simulink model "H9_Heric_2__new_series_switching_upcoming_conference"  (R2018a)
settings: Solver=ode45  StartTime=0.0  StopTime=.04  RelTol=1e-3  EnableMultiTasking=on
libraries: powerlib x53, powerlib_extras x6, powerlib_meascontrol x5, pePowerMeasurement x1, simulink x1
settings Model: Creator=Personal  LastModifiedBy=HP
settings DataIOCC: LimitDataPoints=on  SaveFormat=Array
settings OptimizationCC: LifeSpan=inf
settings DebuggingCC: SolverPrmCheckMsg=warning  SFUnexpectedBacktrackingDiag=warning  SFNoUnconditionalDefaultTransitionDiag=warning  SFExecutionAtInitializationDiag=none
settings HardwareCC: ProdBitPerPointer=32  ProdBitPerSizeT=32  ProdBitPerPtrDiffT=32  ProdLargestAtomicFloat=None  ProdIntDivRoundTo=Undefined  ProdEndianess=Unspecified  ProdWordSize=32  ProdHWDeviceType=32-bit Generic
settings ModelReferenceCC: PropagateSignalLabelsOutOfModel=off
settings CodeAppCC: StateflowObjectComments=on
settings GRTTargetCC: TargetLangStandard=C89/C90 (ANSI)  GeneratePreprocessorConditionals=Disable all
settings ConfigComp: CovMetricSettings=dw  CovHtmlReporting=on  CovSaveCumulativeToWorkspaceVar=on  CovSaveSingleToWorkspaceVar=on  CovExternalEMLEnable=off  CovSFcnEnable=off
settings SimscapeCC: SimscapeNormalizeSystem=off

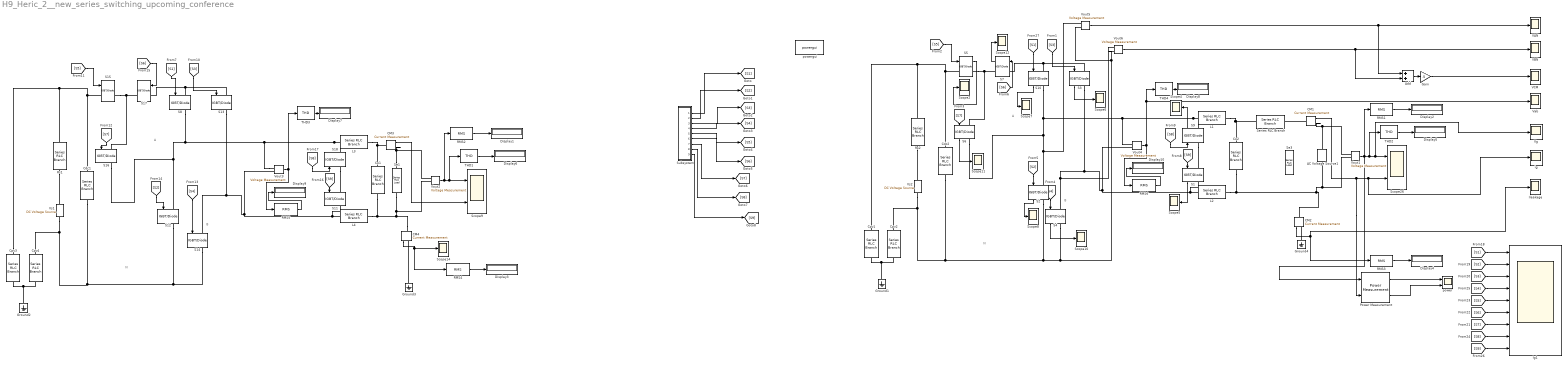
== system H9_Heric_2__new_series_switching_upcoming_conference ==
  note: B
  note: A
  note: N
  note: A
  note: N
  note: B
  AC Voltage Source1 : powerlib/Electrical Sources/AC Voltage Source  Amplitude=220  Phase=0  Frequency=50  SampleTime=0  Measurements=None  BusType=swing  Pref=10e3  Qref=0  Qmin=-inf  Qmax=+inf
  Add : Sum
  CM{1..4} (4 alike) : powerlib/Measurements/Current Measurement  PhasorSimulation=off  OutputType=Complex  PSBequivalent=0
  Cdc1 : powerlib/Elements/Series RLC Branch  LConnTagsString=__new0  RConnTagsString=__new0  BranchType=C  Resistance=1  Inductance=3e-3  SetiL0=off  InitialCurrent=0  Capacitance=940e-6  Setx0=off  InitialVoltage=0  Measurements=None
  Cdc2 : powerlib/Elements/Series RLC Branch  LConnTagsString=__new0  RConnTagsString=__new0  BranchType=C  Resistance=1  Inductance=3e-3  SetiL0=off  InitialCurrent=0  Capacitance=940e-6  Setx0=off  InitialVoltage=0  Measurements=None
  Co1 : powerlib/Elements/Series RLC Branch  LConnTagsString=__new0  RConnTagsString=__new0  BranchType=C  Resistance=1  Inductance=3e-3  SetiL0=off  InitialCurrent=0  Capacitance=2.2e-6  Setx0=off  InitialVoltage=0  Measurements=None
  Co2 : powerlib/Elements/Series RLC Branch  LConnTagsString=__new0  RConnTagsString=__new0  BranchType=C  Resistance=1  Inductance=3e-3  SetiL0=off  InitialCurrent=0  Capacitance=2.2e-6  Setx0=off  InitialVoltage=0  Measurements=None
  Cpv{1..4} (4 alike) : powerlib/Elements/Series RLC Branch  LConnTagsString=__new0  RConnTagsString=__new0  BranchType=C  Resistance=1  Inductance=3e-3  SetiL0=off  InitialCurrent=0  Capacitance=75e-9  Setx0=off  InitialVoltage=0  Measurements=None
  Display{1..10} (10 alike) : Display
  Gain : Gain  Gain=.5
  Ground{1..4} (4 alike) : powerlib/Elements/Ground  LConnTagsString=a
  Ig1 : Scope  NumInputPorts=9
  Ileakage : Scope
  L{1..4} (4 alike) : powerlib/Elements/Series RLC Branch  LConnTagsString=__new0  RConnTagsString=__new0  BranchType=L  Resistance=1  Inductance=3e-3  SetiL0=off  InitialCurrent=0  Capacitance=1e-6  Setx0=off  InitialVoltage=0  Measurements=None
  Power Measurement : pePowerMeasurement/Power Measurement  OverrideUsingVariant=Continuous  F=60  K=[0 1 2 3]  Ts=0
  RMS{1..6} (6 alike) : powerlib_extras/Measurements/RMS  f1=50
  Rs1 : powerlib/Elements/Series RLC Branch  LConnTagsString=__new0  RConnTagsString=__new0  BranchType=R  Resistance=1  Inductance=3e-3  SetiL0=off  InitialCurrent=0  Capacitance=1e-6  Setx0=off  InitialVoltage=0  Measurements=None
  Rs2 : powerlib/Elements/Series RLC Branch  LConnTagsString=__new0  RConnTagsString=__new0  BranchType=R  Resistance=1  Inductance=3e-3  SetiL0=off  InitialCurrent=0  Capacitance=1e-6  Setx0=off  InitialVoltage=0  Measurements=None
  S{1..18} (18 alike) : powerlib/Power Electronics/IGBT//Diode  Ron=1e-3  Rs=1e5  Cs=inf  Measurements=on
  Scope{2,4..8,10..12,14} (10 alike) : Scope
  Scope26 : Scope  NumInputPorts=2
  Scope9 : Scope  NumInputPorts=2
  Se1 : powerlib/Elements/Series RLC Load  LConnTagsString=a  RConnTagsString=__new0  NominalVoltage=230  NominalFrequency=50  ActivePower=1000  InductivePower=0  CapacitivePower=0  Setx0=off  InitialVoltage=0  SetiL0=off  InitialCurrent=0  Measurements=None  LoadType=constant Z
  Se3 : powerlib/Elements/Series RLC Load  LConnTagsString=a  RConnTagsString=__new0  NominalVoltage=230  NominalFrequency=50  ActivePower=1000  InductivePower=0  CapacitivePower=0  Setx0=off  InitialVoltage=0  SetiL0=off  InitialCurrent=0  Measurements=None  LoadType=constant Z
  Series RLC Branch : powerlib/Elements/Series RLC Branch  LConnTagsString=__new0  RConnTagsString=__new0  BranchType=R  Resistance=10  Inductance=1e-3  SetiL0=off  InitialCurrent=0  Capacitance=0  Setx0=off  InitialVoltage=0  Measurements=None
  Subsystem : Subsystem
  THD1 : powerlib_meascontrol/Measurements/THD  Freq=50  Ts=0
  THD2 : powerlib_meascontrol/Measurements/THD  Freq=50  Ts=0
  THD3 : powerlib_meascontrol/Measurements/THD  Freq=60  Ts=0
  THD4 : powerlib_meascontrol/Measurements/THD  Freq=60  Ts=0
  VAN : Scope
  VBN : Scope
  VCM : Scope
  Vab : Scope
  Vg : Scope
  Vout{1..6} (6 alike) : powerlib/Measurements/Voltage Measurement  PhasorSimulation=off  OutputType=Complex  PSBequivalent=0
  Vs1 : powerlib/Electrical Sources/DC Voltage Source  Amplitude=330  Measurements=None
  Vs2 : powerlib/Electrical Sources/DC Voltage Source  Amplitude=330  Measurements=None
  ig : Scope
  power : Scope  NumInputPorts=2
  powergui : powerlib/powergui  Priority=1  SimulationMode=Continuous  SampleTime=50e-6  frequency=60  Iterations=50  frequencyindice=0  Pbase=100e6  ErrMax=1e-4  UnitsV=kV  UnitsW=MW  buscounter=0  FunctionMessages=off  echomessages=off  EnableUseOfTLC=off  CurrentSourceSwitches=off  DisableSnubberDevices=off  DisableRonSwitches=off  DisableVfSwitches=off  DisplayEquations=off  SolverType=Tustin/Backward Euler (TBE)  Interpol=off  ExternalGateDelay=off  methode=off  Ts=100  x0status=blocks  SPID=on  SwTol=0  HookPort=off  RestoreLinks=warning  ResistiveCurrentMeasurement=off  Frange=[0:2:500]  Ylog=off  Xlog=on  ShowGrid=off  save=off  variable=ZData  structure=ig  ZoomFFT=off  StartTime=0.02  cycles=1  DisplayStyle=1  fundamental=50  FreqAxis=off  MaxFrequency=10000  frequencyindicesteady=1  RmsSteady=1  display=off
  wires:
  Subsystem/1(Out1) -> [S1]
  Subsystem/2(Out2) -> [S2]
  Subsystem/3(Out3) -> [S3]
  Subsystem/4(Out4) -> [S4]
  Subsystem/5(Out5) -> [S5]
  Subsystem/6(Out6) -> [S6]
  Subsystem/7(Out7) -> [S7]
  Subsystem/8(Out8) -> [S8]
  Subsystem/9(Out9) -> [S9]
  ? -> ?
  [S5] -> S15/1
  [S8] -> S18/1
  [S6] -> S17/1
  [S9] -> S11/1
  CM3/1 -> Scope9/2
  CM4/1 -> Scope14/1, RMS4/1
  [S7] -> S16/1
  RMS4/1 -> Display3/1
  [S1] -> S8/1
  THD3/1 -> Display7/1
  [S2] -> S12/1
  Vout2/1 -> RMS2/1, THD1/1, Scope9/1
  THD1/1 -> Display6/1
  [S4] -> S14/1
  RMS5/1 -> Display9/1
  RMS2/1 -> Display1/1
  [S3] -> S13/1
  Vout3/1 -> THD3/1, RMS5/1
  [S4] -> Ig1/4
  [S6] -> Ig1/6
  [S5] -> Ig1/5
  [S7] -> Ig1/7
  [S1] -> Ig1/1
  [S3] -> Ig1/3
  [S2] -> Ig1/2
  [S8] -> Ig1/8
  [S9] -> Ig1/9
  RMS6/1 -> Display10/1
  RMS1/1 -> Display2/1
  [S4] -> S4/1
  [S7] -> S6/1
  [S1] -> S10/1
  S3/1 -> Scope6/1
  [S2] -> S2/1
  THD2/1 -> Display5/1
  S2/1 -> Scope8/1
  S9/1 -> Scope4/1
  RMS3/1 -> Display4/1
  Vout4/1 -> THD4/1, Vab/1, RMS6/1
  S6/1 -> Scope11/1
  [S3] -> S3/1
  S10/1 -> Scope7/1
  [S8] -> S9/1
  [S5] -> S5/1
  [S6] -> S7/1
  [S9] -> S1/1
  THD4/1 -> Display8/1
  S7/1 -> Scope12/1
  CM2/1 -> Ileakage/1, RMS3/1
  S4/1 -> Scope10/1
  S5/1 -> Scope2/1
  S1/1 -> Scope5/1
  Vout6/1 -> Add/2, VBN/1
  Vout5/1 -> Add/1, VAN/1
  Add/1 -> Gain/1
  Gain/1 -> VCM/1
  Power Measurement/1 -> power/1
  Vout1/1 -> Scope26/1, Vg/1, THD2/1, RMS1/1, Power Measurement/1
  Power Measurement/2 -> power/2
  CM1/1 -> Power Measurement/2, ig/1, Scope26/2
  connections:
  S12/RConn1 -- S14/RConn1 -- Vs1/LConn1 -- Cpv4/LConn1 -- Cdc1/RConn1
  S17/LConn1 -- S13/LConn1 -- S8/LConn1
  S13/RConn1 -- Vout3/LConn2 -- L4/LConn1 -- S11/RConn1 -- S14/LConn1
  CM4/LConn1 -- Vout2/LConn2 -- Se1/RConn1 -- L4/RConn1 -- Co1/RConn1
  Cpv3/LConn1 -- Cdc1/LConn1 -- S15/LConn1 -- Rs1/RConn1
  Vout3/LConn1 -- S16/RConn1 -- S12/LConn1 -- S8/RConn1 -- L3/LConn1 -- S18/RConn1
  Co1/LConn1 -- L3/RConn1 -- CM3/LConn1
  S16/LConn1 -- S15/RConn1 -- S17/RConn1
  Cpv3/RConn1 -- Ground2/LConn1 -- Cpv4/RConn1
  Se1/LConn1 -- CM3/RConn1 -- Vout2/LConn1
  Ground3/LConn1 -- CM4/RConn1
  Rs1/LConn1 -- Vs1/RConn1
  S18/LConn1 -- S11/LConn1
  S9/RConn1 -- Vout4/LConn1 -- S6/RConn1 -- S2/LConn1 -- Vout5/LConn1 -- S10/RConn1 -- L1/LConn1
  Cpv2/RConn1 -- Cpv1/RConn1 -- Ground1/LConn1
  Vout1/LConn2 -- CM2/LConn1 -- L2/RConn1 -- Co2/RConn1 -- AC Voltage Source1/LConn1
  S5/LConn1 -- Cpv1/LConn1 -- Rs2/RConn1 -- Cdc2/LConn1
  S10/LConn1 -- S7/LConn1 -- S3/LConn1
  S4/RConn1 -- Vout6/LConn2 -- Vout5/LConn2 -- Vs2/LConn1 -- Cpv2/LConn1 -- Cdc2/RConn1 -- S2/RConn1
  S1/RConn1 -- S4/LConn1 -- Vout6/LConn1 -- S3/RConn1 -- Vout4/LConn2 -- L2/LConn1
  CM1/LConn1 -- Series RLC Branch/RConn1
  Vout1/LConn1 -- CM1/RConn1 -- AC Voltage Source1/RConn1
  S7/RConn1 -- S6/LConn1 -- S5/RConn1
  Ground4/LConn1 -- CM2/RConn1
  Rs2/LConn1 -- Vs2/RConn1
  S9/LConn1 -- S1/LConn1
  Series RLC Branch/LConn1 -- Co2/LConn1 -- L1/RConn1

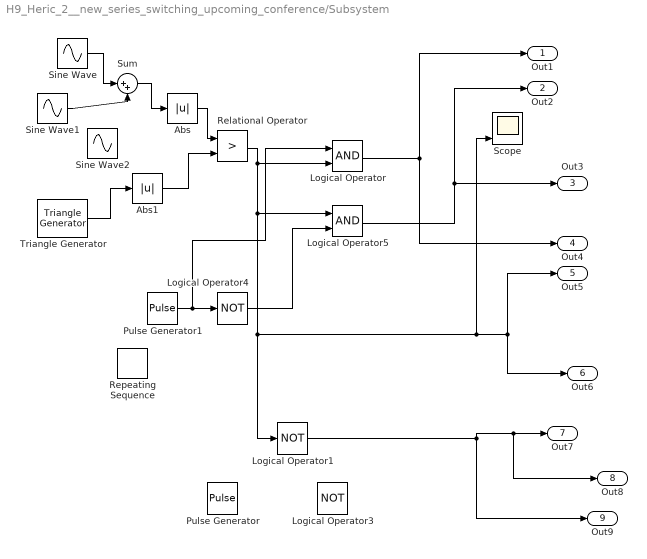
== system H9_Heric_2__new_series_switching_upcoming_conference/Subsystem ==
  Abs : Abs
  Abs1 : Abs
  Logical Operator : Logic  AllPortsSameDT=off  OutDataTypeStr=boolean
  Logical Operator1 : Logic  Operator=NOT  AllPortsSameDT=off  OutDataTypeStr=boolean
  Logical Operator3 : Logic  Operator=NOT  AllPortsSameDT=off  OutDataTypeStr=boolean
  Logical Operator4 : Logic  Operator=NOT  AllPortsSameDT=off  OutDataTypeStr=boolean
  Logical Operator5 : Logic  AllPortsSameDT=off  OutDataTypeStr=boolean
  Pulse Generator : DiscretePulseGenerator  PulseType=Time based  Period=.02  PulseWidth=50
  Pulse Generator1 : DiscretePulseGenerator  PulseType=Time based  Period=.02  PulseWidth=50
  Relational Operator : RelationalOperator  Operator=>  OutDataTypeStr=boolean  RndMeth=Nearest
  Repeating Sequence : simulink/Sources/Repeating Sequence  rep_seq_t=[0 1]*(1/20000)  rep_seq_y=[0 1]
  Scope : Scope  NumInputPorts=3
  Sine Wave : Sin  Frequency=2*pi*50  SampleTime=0
  Sine Wave1 : Sin  Amplitude=.003  Frequency=2*pi*3*50  Phase=pi  SampleTime=0
  Sine Wave2 : Sin  Amplitude=.001  Frequency=2*pi*5*50  Phase=pi  SampleTime=0
  Sum : Sum  Inputs=|++
  Triangle Generator : powerlib_meascontrol/Pulse & Signal Generators/Triangle Generator  Freq=8e3  Phase=90  Ts=0
  Out1 : Outport
  Out2 : Outport  Port=2
  Out3 : Outport  Port=3
  Out4 : Outport  Port=4
  Out5 : Outport  Port=5
  Out6 : Outport  Port=6
  Out7 : Outport  Port=7
  Out8 : Outport  Port=8
  Out9 : Outport  Port=9
  wires:
  Triangle Generator/1 -> Abs1/1
  Relational Operator/1 -> Logical Operator1/1, Out6/1, Out5/1, Scope/3, Logical Operator5/1, Logical Operator/2
  Abs1/1 -> Relational Operator/2
  Abs/1 -> Relational Operator/1
  Sine Wave/1 -> Sum/1
  Sum/1 -> Abs/1
  Pulse Generator1/1 -> Logical Operator/1, Logical Operator4/1
  Logical Operator4/1 -> Logical Operator5/2
  Logical Operator1/1 -> Out8/1, Out7/1, Out9/1
  Sine Wave1/1 -> Sum/2
  Logical Operator/1 -> Out1/1, Out4/1
  Logical Operator5/1 -> Out2/1, Out3/1
